simulink library "IO"  (R2025a)
settings: Solver=VariableStepAuto  StartTime=0.0  StopTime=10.0  RelTol=1e-3
values from neighbouring files (symbols this model uses):
  ADCBits = 12.0    [IO.sldd]
  Vref = 5.0    [IO.sldd]
undefined symbols (not defined in the file or in its folder): Bridge, dt, H, raptor_xcp_function
libraries: Raptor_lib x133, Utilities x20, Cooling x1
(part 2 of 6)

== system IO/CANOutputs/TCRegen ==
  IO_CAN2_154_Bus : Inport
  Bus Selector : BusSelector  OutputSignals=IO_RegenEnable_en,IO_TCActive_bool,IO_TCEnable_en,IO_TCSensitivity_en
  RollingCounterGenerator : Utilities/RollingCounterGenerator
  raptor_can_txmsg : Raptor_lib/CAN/raptor_can_txmsg  canDefinition=struct('dbcFile', 'SR26_CAN2.dbc','message', 'VCU_154','comment', '','signals', {{'VCU_counterMsg154','VCU_regenEnable','VCU_tCActive','VCU_tCEnable','VCU_tCSensitivity'}},'enabled', [ 1 1 1 1 1;],'scaled', [ 1 1 1 1 1;],'canBus', '''CAN2''','messageID', [ 154;],'idMask', [ 536870911;],'payloadMask', [],'payloadValue', [],'useDbcPeriod', [ 0;],'period', [ 100;],'queueSize', [ 1;],'label', [ 0;],'ver', [ 2;],'showID', [ 0;],'showRaw', [ 0;],'showRawMsg', [ 0;],'useStartVals', [ 0;],'extendedId', [ 0;],'useSimFunc', [ 0;],'sim_func_name', '''''','fill', [ 0;],'editID', [ 0;],'signalOrder', [ 1;],'signalAscDes', [ 1;],'msgLength', [ 8;])  canBus='CAN2'  queueSize=1  payloadMask=[]  payloadValue=[]  period=100  showID=0  label=0  idMask=hex2dec('1FFFFFFF')  fill=0  id=154  showRaw=0  signalOrder=1  signalInfo={{struct('Name', 'VCU_regenEnable','StartBit', [ 48;],'SignalSize', [ 8;],'ByteOrder', 'LittleEndian','ValueType', 'UNSIGNED','Class', 'uint8','Signed', [ 0;],'Factor', [ 1;],'Offset', [ 0;],'Min', [ 0;],'Max', [ 255;],'Units', '','StartVal', [ 0;],'Comment', 'Enumeration','Multiplexed', [ 0;],'Multiplexor', [ 0;],'MultiplexMode_Min', [],'MultiplexMode_Max', []),struct('Name', 'VCU_tCEnable','StartBit', [ 40;],'SignalSize', [ 8;],'ByteOrder', 'LittleEndian','ValueType', 'UNSIGNED','Class', 'uint8','Signed', [ 0;],'Factor', [ 1;],'Offset', [ 0;],'Min', [ 0;],'Max', [ 255;],'Units', '','StartVal', [ 0;],'Comment', 'Enumeration','Multiplexed', [ 0;],'Multiplexor', [ 0;],'MultiplexMode_Min', [],'MultiplexMode_Max', []),struct('Name', 'VCU_tCActive','StartBit', [ 32;],'SignalSize', [ 8;],'ByteOrder', 'LittleEndian','ValueType', 'UNSIGNED','Class', 'uint8','Signed', [ 0;],'Factor', [ 1;],'Offset', [ 0;],'Min', [ 0;],'Max', [ 255;],'Units', '','StartVal', [ 0;],'Comment', '0 = off, 1 = on Enumeration','Multiplexed', [ 0;],'Multiplexor', [ 0;],'MultiplexMode_Min', [],'MultiplexMode_Max', []),struct('Name', 'VCU_tCSensitivity','StartBit', [ 16;],'SignalSize', [ 16;],'ByteOrder', 'LittleEndian','ValueType', 'UNSIGNED','Class', 'uint16','Signed', [ 0;],'Factor', [ 1;],'Offset', [ 0;],'Min', [ -20;],'Max', [ 3276.7;],'Units', '','StartVal', [ 0;],'Comment', '','Multiplexed', [ 0;],'Multiplexor', [ 0;],'MultiplexMode_Min', [],'MultiplexMode_Max', []),struct('Name', 'VCU_counterMsg154','StartBit', [ 0;],'SignalSize', [ 4;],'ByteOrder', 'LittleEndian','ValueType', 'UNSIGNED','Class', 'uint8','Signed', [ 0;],'Factor', [ 1;],'Offset', [ 0;],'Min', [ 0;],'Max', [ 15;],'Units', '','StartVal', [ 0;],'Comment', 'Counter Message 154','Multiplexed', [ 0;],'Multiplexor', [ 0;],'MultiplexMode_Min', [],'MultiplexMode_Max', [])}}  useSimFunc=0  sim_func_name=''  useStartVals=0
      settings: SourceProductName=Raptor
  raptor_function_call_collector : Raptor_lib/Triggers/raptor_function_call_collector  count=10
      settings: SourceProductName=Raptor
  wires:
  Bus Selector/4 -> raptor_can_txmsg/5  "<IO_TCSensitivity_en>"
  Bus Selector/3 -> raptor_can_txmsg/4  "<IO_TCEnable_en>"
  Bus Selector/2 -> raptor_can_txmsg/3  "<IO_TCActive_bool>"
  Bus Selector/1 -> raptor_can_txmsg/2  "<IO_RegenEnable_en>"
  IO_CAN2_154_Bus/1 -> Bus Selector/1
  raptor_function_call_collector/1 -> RollingCounterGenerator/Trigger
  RollingCounterGenerator/1 -> raptor_can_txmsg/1

== system IO/CANOutputs/Throttle ==
  IO_CAN2_150_Bus : Inport
  Bus Selector : BusSelector  OutputSignals=IO_ThrottlePosition_pct,IO_ThrottlePosition1_pct,IO_ThrottlePosition2_pct
  RollingCounterGenerator : Utilities/RollingCounterGenerator
  raptor_can_txmsg : Raptor_lib/CAN/raptor_can_txmsg  canDefinition=struct('dbcFile', 'SR26_CAN2.dbc','message', 'VCU_150','comment', '','signals', {{'VCU_counterMsg150','VCU_throttlePosition','VCU_throttlePosition1','VCU_throttlePosition2'}},'enabled', [ 1 1 1 1;],'scaled', [ 1 1 1 1;],'canBus', '''CAN2''','messageID', [ 150;],'idMask', [ 536870911;],'payloadMask', [],'payloadValue', [],'useDbcPeriod', [ 0;],'period', [ 100;],'queueSize', [ 1;],'label', [ 0;],'ver', [ 2;],'showID', [ 0;],'showRaw', [ 0;],'showRawMsg', [ 0;],'useStartVals', [ 0;],'extendedId', [ 0;],'useSimFunc', [ 0;],'sim_func_name', '''''','fill', [ 0;],'editID', [ 0;],'signalOrder', [ 1;],'signalAscDes', [ 1;],'msgLength', [ 8;])  canBus='CAN2'  queueSize=1  payloadMask=[]  payloadValue=[]  period=100  showID=0  label=0  idMask=hex2dec('1FFFFFFF')  fill=0  id=150  showRaw=0  signalOrder=1  signalInfo={{struct('Name', 'VCU_throttlePosition2','StartBit', [ 48;],'SignalSize', [ 16;],'ByteOrder', 'LittleEndian','ValueType', 'SIGNED','Class', 'int16','Signed', [ 1;],'Factor', [ 0.1;],'Offset', [ 0;],'Min', [ 0;],'Max', [ 100;],'Units', '%','StartVal', [ 0;],'Comment', 'TPS2','Multiplexed', [ 0;],'Multiplexor', [ 0;],'MultiplexMode_Min', [],'MultiplexMode_Max', []),struct('Name', 'VCU_throttlePosition1','StartBit', [ 32;],'SignalSize', [ 16;],'ByteOrder', 'LittleEndian','ValueType', 'SIGNED','Class', 'int16','Signed', [ 1;],'Factor', [ 0.1;],'Offset', [ 0;],'Min', [ 0;],'Max', [ 100;],'Units', '%','StartVal', [ 0;],'Comment', 'TPS1','Multiplexed', [ 0;],'Multiplexor', [ 0;],'MultiplexMode_Min', [],'MultiplexMode_Max', []),struct('Name', 'VCU_throttlePosition','StartBit', [ 16;],'SignalSize', [ 16;],'ByteOrder', 'LittleEndian','ValueType', 'SIGNED','Class', 'int16','Signed', [ 1;],'Factor', [ 0.1;],'Offset', [ 0;],'Min', [ 0;],'Max', [ 100;],'Units', '%','StartVal', [ 0;],'Comment', 'Final throttle position','Multiplexed', [ 0;],'Multiplexor', [ 0;],'MultiplexMode_Min', [],'MultiplexMode_Max', []),struct('Name', 'VCU_counterMsg150','StartBit', [ 0;],'SignalSize', [ 4;],'ByteOrder', 'LittleEndian','ValueType', 'UNSIGNED','Class', 'uint8','Signed', [ 0;],'Factor', [ 1;],'Offset', [ 0;],'Min', [ 0;],'Max', [ 15;],'Units', '','StartVal', [ 0;],'Comment', 'Counter Message 150','Multiplexed', [ 0;],'Multiplexor', [ 0;],'MultiplexMode_Min', [],'MultiplexMode_Max', [])}}  useSimFunc=0  sim_func_name=''  useStartVals=0
      settings: SourceProductName=Raptor
  raptor_function_call_collector : Raptor_lib/Triggers/raptor_function_call_collector  count=10
      settings: SourceProductName=Raptor
  wires:
  IO_CAN2_150_Bus/1 -> Bus Selector/1
  Bus Selector/1 -> raptor_can_txmsg/2  "<IO_ThrottlePosition_pct>"
  Bus Selector/2 -> raptor_can_txmsg/3  "<IO_ThrottlePosition1_pct>"
  Bus Selector/3 -> raptor_can_txmsg/4  "<IO_ThrottlePosition2_pct>"
  RollingCounterGenerator/1 -> raptor_can_txmsg/1
  raptor_function_call_collector/1 -> RollingCounterGenerator/Trigger

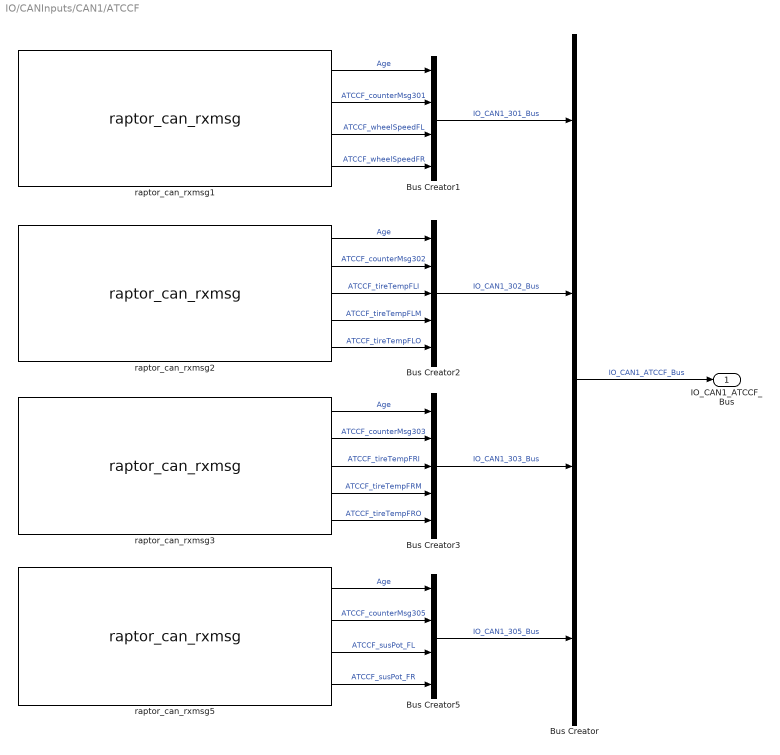
== system IO/CANInputs/CAN1/ATCCF ==
  Bus Creator : BusCreator  Inputs=4
  Bus Creator1 : BusCreator  Inputs=4
  Bus Creator2 : BusCreator  Inputs=5
  Bus Creator3 : BusCreator  Inputs=5
  Bus Creator5 : BusCreator  Inputs=4
  raptor_can_rxmsg1 : Raptor_lib/CAN/raptor_can_rxmsg  canDefinition=struct('dbcFile', 'SR26_CAN1.dbc','message', 'ATCCF_301','comment', '','signals', {{'ATCCF_counterMsg301','ATCCF_wheelSpeedFL','ATCCF_wheelSpeedFR'}},'enabled', [ 1 1 1;],'scaled', [ 1 1 1;],'canBus', '''CAN1''','messageID', [ 301;],'idMask', [ 536870911;],'payloadMask', [],'payloadValue', [],'period', [ 0;],'mailbox', '''''','queueSize', [ 1;],'label', [ 0;],'ver', [ 2;],'showID', [ 0;],'showRaw', [ 0;],'showRawMsg', [ 0;],'useStartVals', [ 0;],'extendedId', [ 0;],'showAge', [ 1;],'useSimFunc', [ 0;],'sim_func_name', '''''','fill', [ 0;],'editID', [ 0;],'signalOrder', [ 1;],'signalAscDes', [ 1;],'msgLength', [ 8;])  canBus='CAN1'  mailbox=''  payloadMask=[]  payloadValue=[]  idMask=hex2dec('1FFFFFFF')  queueSize=1  showID=0  label=0  fill=0  id=301  showRaw=0  showAge=1  signalOrder=1  signalInfo={{struct('Name', 'ATCCF_wheelSpeedFR','StartBit', [ 32;],'SignalSize', [ 16;],'ByteOrder', 'LittleEndian','ValueType', 'UNSIGNED','Class', 'uint16','Signed', [ 0;],'Factor', [ 1;],'Offset', [ 0;],'Min', [ 0;],'Max', [ 2000;],'Units', 'Hz','StartVal', [ 0;],'Comment', 'FR Angular Wheel Frequency','Multiplexed', [ 0;],'Multiplexor', [ 0;],'MultiplexMode_Min', [],'MultiplexMode_Max', []),struct('Name', 'ATCCF_wheelSpeedFL','StartBit', [ 16;],'SignalSize', [ 16;],'ByteOrder', 'LittleEndian','ValueType', 'UNSIGNED','Class', 'uint16','Signed', [ 0;],'Factor', [ 1;],'Offset', [ 0;],'Min', [ 0;],'Max', [ 2000;],'Units', 'Hz','StartVal', [ 0;],'Comment', 'FL Angular Wheel Frequency','Multiplexed', [ 0;],'Multiplexor', [ 0;],'MultiplexMode_Min', [],'MultiplexMode_Max', []),struct('Name', 'ATCCF_counterMsg301','StartBit', [ 0;],'SignalSize', [ 4;],'ByteOrder', 'LittleEndian','ValueType', 'UNSIGNED','Class', 'uint8','Signed', [ 0;],'Factor', [ 1;],'Offset', [ 0;],'Min', [ 0;],'Max', [ 15;],'Units', '','StartVal', [ 0;],'Comment', 'Counter Message 301','Multiplexed', [ 0;],'Multiplexor', [ 0;],'MultiplexMode_Min', [],'MultiplexMode_Max', [])}}  showRawMsg=0  useSimFunc=0  sim_func_name=''  useStartVals=0  extendedId=0
      settings: SourceProductName=Raptor
  raptor_can_rxmsg2 : Raptor_lib/CAN/raptor_can_rxmsg  canDefinition=struct('dbcFile', 'SR26_CAN1.dbc','message', 'ATCCF_302','comment', '','signals', {{'ATCCF_counterMsg302','ATCCF_tireTemp_FLI','ATCCF_tireTemp_FLM','ATCCF_tireTemp_FLO'}},'enabled', [ 1 1 1 1;],'scaled', [ 1 1 1 1;],'canBus', '''CAN1''','messageID', [ 302;],'idMask', [ 536870911;],'payloadMask', [],'payloadValue', [],'period', [ 0;],'mailbox', '''''','queueSize', [ 1;],'label', [ 0;],'ver', [ 2;],'showID', [ 0;],'showRaw', [ 0;],'showRawMsg', [ 0;],'useStartVals', [ 0;],'extendedId', [ 0;],'showAge', [ 1;],'useSimFunc', [ 0;],'sim_func_name', '''''','fill', [ 0;],'editID', [ 0;],'signalOrder', [ 1;],'signalAscDes', [ 1;],'msgLength', [ 8;])  canBus='CAN1'  mailbox=''  payloadMask=[]  payloadValue=[]  idMask=hex2dec('1FFFFFFF')  queueSize=1  showID=0  label=0  fill=0  id=302  showRaw=0  showAge=1  signalOrder=1  signalInfo={{struct('Name', 'ATCCF_tireTemp_FLI','StartBit', [ 48;],'SignalSize', [ 16;],'ByteOrder', 'LittleEndian','ValueType', 'SIGNED','Class', 'int16','Signed', [ 1;],'Factor', [ 1;],'Offset', [ 0;],'Min', [ 0;],'Max', [ 150;],'Units', 'degC','StartVal', [ 0;],'Comment', '','Multiplexed', [ 0;],'Multiplexor', [ 0;],'MultiplexMode_Min', [],'MultiplexMode_Max', []),struct('Name', 'ATCCF_tireTemp_FLM','StartBit', [ 32;],'SignalSize', [ 16;],'ByteOrder', 'LittleEndian','ValueType', 'SIGNED','Class', 'int16','Signed', [ 1;],'Factor', [ 1;],'Offset', [ 0;],'Min', [ 0;],'Max', [ 150;],'Units', 'degC','StartVal', [ 0;],'Comment', '','Multiplexed', [ 0;],'Multiplexor', [ 0;],'MultiplexMode_Min', [],'MultiplexMode_Max', []),struct('Name', 'ATCCF_tireTemp_FLO','StartBit', [ 16;],'SignalSize', [ 16;],'ByteOrder', 'LittleEndian','ValueType', 'SIGNED','Class', 'int16','Signed', [ 1;],'Factor', [ 1;],'Offset', [ 0;],'Min', [ 0;],'Max', [ 150;],'Units', 'degC','StartVal', [ 0;],'Comment', '','Multiplexed', [ 0;],'Multiplexor', [ 0;],'MultiplexMode_Min', [],'MultiplexMode_Max', []),struct('Name', 'ATCCF_counterMsg302','StartBit', [ 0;],'SignalSize', [ 4;],'ByteOrder', 'LittleEndian','ValueType', 'UNSIGNED','Class', 'uint8','Signed', [ 0;],'Factor', [ 1;],'Offset', [ 0;],'Min', [ 0;],'Max', [ 15;],'Units', '','StartVal', [ 0;],'Comment', '','Multiplexed', [ 0;],'Multiplexor', [ 0;],'MultiplexMode_Min', [],'MultiplexMode_Max', [])}}  showRawMsg=0  useSimFunc=0  sim_func_name=''  useStartVals=0  extendedId=0
      settings: SourceProductName=Raptor
  raptor_can_rxmsg3 : Raptor_lib/CAN/raptor_can_rxmsg  canDefinition=struct('dbcFile', 'SR26_CAN1.dbc','message', 'ATCCF_303','comment', '','signals', {{'ATCCF_counterMsg303','ATCCF_tireTemp_FRI','ATCCF_tireTemp_FRM','ATCCF_tireTemp_FRO'}},'enabled', [ 1 1 1 1;],'scaled', [ 1 1 1 1;],'canBus', '''CAN1''','messageID', [ 303;],'idMask', [ 536870911;],'payloadMask', [],'payloadValue', [],'period', [ 0;],'mailbox', '''''','queueSize', [ 1;],'label', [ 0;],'ver', [ 2;],'showID', [ 0;],'showRaw', [ 0;],'showRawMsg', [ 0;],'useStartVals', [ 0;],'extendedId', [ 0;],'showAge', [ 1;],'useSimFunc', [ 0;],'sim_func_name', '''''','fill', [ 0;],'editID', [ 0;],'signalOrder', [ 1;],'signalAscDes', [ 1;],'msgLength', [ 8;])  canBus='CAN1'  mailbox=''  payloadMask=[]  payloadValue=[]  idMask=hex2dec('1FFFFFFF')  queueSize=1  showID=0  label=0  fill=0  id=303  showRaw=0  showAge=1  signalOrder=1  signalInfo={{struct('Name', 'ATCCF_tireTemp_FRI','StartBit', [ 48;],'SignalSize', [ 16;],'ByteOrder', 'LittleEndian','ValueType', 'SIGNED','Class', 'int16','Signed', [ 1;],'Factor', [ 1;],'Offset', [ 0;],'Min', [ 0;],'Max', [ 150;],'Units', 'degC','StartVal', [ 0;],'Comment', '','Multiplexed', [ 0;],'Multiplexor', [ 0;],'MultiplexMode_Min', [],'MultiplexMode_Max', []),struct('Name', 'ATCCF_tireTemp_FRM','StartBit', [ 32;],'SignalSize', [ 16;],'ByteOrder', 'LittleEndian','ValueType', 'SIGNED','Class', 'int16','Signed', [ 1;],'Factor', [ 1;],'Offset', [ 0;],'Min', [ 0;],'Max', [ 150;],'Units', 'degC','StartVal', [ 0;],'Comment', '','Multiplexed', [ 0;],'Multiplexor', [ 0;],'MultiplexMode_Min', [],'MultiplexMode_Max', []),struct('Name', 'ATCCF_tireTemp_FRO','StartBit', [ 16;],'SignalSize', [ 16;],'ByteOrder', 'LittleEndian','ValueType', 'SIGNED','Class', 'int16','Signed', [ 1;],'Factor', [ 1;],'Offset', [ 0;],'Min', [ 0;],'Max', [ 150;],'Units', 'degC','StartVal', [ 0;],'Comment', '','Multiplexed', [ 0;],'Multiplexor', [ 0;],'MultiplexMode_Min', [],'MultiplexMode_Max', []),struct('Name', 'ATCCF_counterMsg303','StartBit', [ 0;],'SignalSize', [ 4;],'ByteOrder', 'LittleEndian','ValueType', 'UNSIGNED','Class', 'uint8','Signed', [ 0;],'Factor', [ 1;],'Offset', [ 0;],'Min', [ 0;],'Max', [ 15;],'Units', '','StartVal', [ 0;],'Comment', '','Multiplexed', [ 0;],'Multiplexor', [ 0;],'MultiplexMode_Min', [],'MultiplexMode_Max', [])}}  showRawMsg=0  useSimFunc=0  sim_func_name=''  useStartVals=0  extendedId=0
      settings: SourceProductName=Raptor
  raptor_can_rxmsg5 : Raptor_lib/CAN/raptor_can_rxmsg  canDefinition=struct('dbcFile', 'SR26_CAN1.dbc','message', 'ATCCF_305','comment', '','signals', {{'ATCCF_counterMsg305','ATCCF_susPot_FL','ATCCF_susPot_FR'}},'enabled', [ 1 1 1;],'scaled', [ 1 1 1;],'canBus', '''CAN1''','messageID', [ 305;],'idMask', [ 536870911;],'payloadMask', [],'payloadValue', [],'period', [ 0;],'mailbox', '''''','queueSize', [ 1;],'label', [ 0;],'ver', [ 2;],'showID', [ 0;],'showRaw', [ 0;],'showRawMsg', [ 0;],'useStartVals', [ 0;],'extendedId', [ 0;],'showAge', [ 1;],'useSimFunc', [ 0;],'sim_func_name', '''''','fill', [ 0;],'editID', [ 0;],'signalOrder', [ 1;],'signalAscDes', [ 1;],'msgLength', [ 8;])  canBus='CAN1'  mailbox=''  payloadMask=[]  payloadValue=[]  idMask=hex2dec('1FFFFFFF')  queueSize=1  showID=0  label=0  fill=0  id=305  showRaw=0  showAge=1  signalOrder=1  signalInfo={{struct('Name', 'ATCCF_susPot_FL','StartBit', [ 32;],'SignalSize', [ 16;],'ByteOrder', 'LittleEndian','ValueType', 'SIGNED','Class', 'int16','Signed', [ 1;],'Factor', [ 1;],'Offset', [ 0;],'Min', [ 0;],'Max', [ 500;],'Units', 'degC','StartVal', [ 0;],'Comment', '','Multiplexed', [ 0;],'Multiplexor', [ 0;],'MultiplexMode_Min', [],'MultiplexMode_Max', []),struct('Name', 'ATCCF_susPot_FR','StartBit', [ 16;],'SignalSize', [ 16;],'ByteOrder', 'LittleEndian','ValueType', 'SIGNED','Class', 'int16','Signed', [ 1;],'Factor', [ 1;],'Offset', [ 0;],'Min', [ 0;],'Max', [ 500;],'Units', 'degC','StartVal', [ 0;],'Comment', '','Multiplexed', [ 0;],'Multiplexor', [ 0;],'MultiplexMode_Min', [],'MultiplexMode_Max', []),struct('Name', 'ATCCF_counterMsg305','StartBit', [ 0;],'SignalSize', [ 4;],'ByteOrder', 'LittleEndian','ValueType', 'UNSIGNED','Class', 'uint8','Signed', [ 0;],'Factor', [ 1;],'Offset', [ 0;],'Min', [ 0;],'Max', [ 15;],'Units', '','StartVal', [ 0;],'Comment', '','Multiplexed', [ 0;],'Multiplexor', [ 0;],'MultiplexMode_Min', [],'MultiplexMode_Max', [])}}  showRawMsg=0  useSimFunc=0  sim_func_name=''  useStartVals=0  extendedId=0
      settings: SourceProductName=Raptor
  IO_CAN1_ATCCF_Bus : Outport
  wires:
  Bus Creator/1 -> IO_CAN1_ATCCF_Bus/1  "IO_CAN1_ATCCF_Bus"
  raptor_can_rxmsg5/1 -> Bus Creator5/1  "Age"
  raptor_can_rxmsg5/2 -> Bus Creator5/2  "ATCCF_counterMsg305"
  raptor_can_rxmsg5/3 -> Bus Creator5/3  "ATCCF_susPot_FL"
  raptor_can_rxmsg5/4 -> Bus Creator5/4  "ATCCF_susPot_FR"
  Bus Creator5/1 -> Bus Creator/4  "IO_CAN1_305_Bus"
  raptor_can_rxmsg3/1 -> Bus Creator3/1  "Age"
  raptor_can_rxmsg3/2 -> Bus Creator3/2  "ATCCF_counterMsg303"
  raptor_can_rxmsg3/3 -> Bus Creator3/3  "ATCCF_tireTempFRI"
  raptor_can_rxmsg3/4 -> Bus Creator3/4  "ATCCF_tireTempFRM"
  Bus Creator3/1 -> Bus Creator/3  "IO_CAN1_303_Bus"
  raptor_can_rxmsg3/5 -> Bus Creator3/5  "ATCCF_tireTempFRO"
  raptor_can_rxmsg2/5 -> Bus Creator2/5  "ATCCF_tireTempFLO"
  Bus Creator2/1 -> Bus Creator/2  "IO_CAN1_302_Bus"
  raptor_can_rxmsg2/4 -> Bus Creator2/4  "ATCCF_tireTempFLM"
  raptor_can_rxmsg2/3 -> Bus Creator2/3  "ATCCF_tireTempFLI"
  raptor_can_rxmsg2/2 -> Bus Creator2/2  "ATCCF_counterMsg302"
  raptor_can_rxmsg2/1 -> Bus Creator2/1  "Age"
  raptor_can_rxmsg1/1 -> Bus Creator1/1  "Age"
  raptor_can_rxmsg1/2 -> Bus Creator1/2  "ATCCF_counterMsg301"
  raptor_can_rxmsg1/3 -> Bus Creator1/3  "ATCCF_wheelSpeedFL"
  raptor_can_rxmsg1/4 -> Bus Creator1/4  "ATCCF_wheelSpeedFR"
  Bus Creator1/1 -> Bus Creator/1  "IO_CAN1_301_Bus"

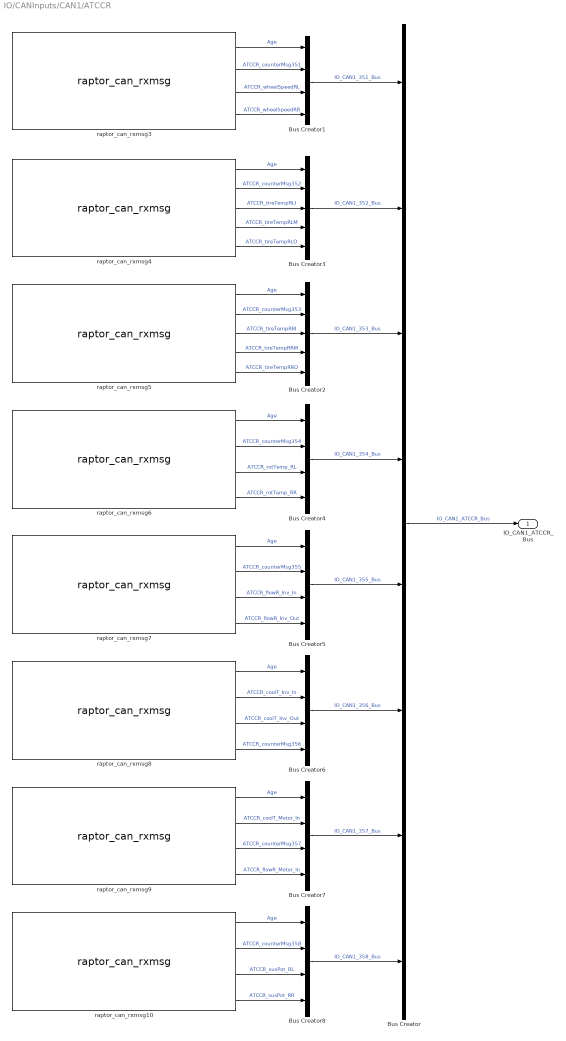
== system IO/CANInputs/CAN1/ATCCR ==
  Bus Creator : BusCreator  Inputs=8
  Bus Creator{1,4..8} (6 alike) : BusCreator  Inputs=4
  Bus Creator2 : BusCreator  Inputs=5
  Bus Creator3 : BusCreator  Inputs=5
  raptor_can_rxmsg10 : Raptor_lib/CAN/raptor_can_rxmsg  canDefinition=struct('dbcFile', 'SR26_CAN1.dbc','message', 'ATCCR_358','comment', '','signals', {{'ATCCR_counterMsg358','ATCCR_susPot_RL','ATCCR_susPot_RR'}},'enabled', [ 1 1 1;],'scaled', [ 1 1 1;],'canBus', '''CAN1''','messageID', [ 358;],'idMask', [ 536870911;],'payloadMask', [],'payloadValue', [],'period', [ 0;],'mailbox', '''''','queueSize', [ 1;],'label', [ 0;],'ver', [ 2;],'showID', [ 0;],'showRaw', [ 0;],'showRawMsg', [ 0;],'useStartVals', [ 0;],'extendedId', [ 0;],'showAge', [ 1;],'useSimFunc', [ 0;],'sim_func_name', '''''','fill', [ 0;],'editID', [ 0;],'signalOrder', [ 1;],'signalAscDes', [ 1;],'msgLength', [ 8;])  canBus='CAN1'  mailbox=''  payloadMask=[]  payloadValue=[]  idMask=hex2dec('1FFFFFFF')  queueSize=1  showID=0  label=0  fill=0  id=358  showRaw=0  showAge=1  signalOrder=1  signalInfo={{struct('Name', 'ATCCR_susPot_RR','StartBit', [ 32;],'SignalSize', [ 16;],'ByteOrder', 'LittleEndian','ValueType', 'SIGNED','Class', 'int16','Signed', [ 1;],'Factor', [ 1;],'Offset', [ 0;],'Min', [ 0;],'Max', [ 500;],'Units', 'degC','StartVal', [ 0;],'Comment', '','Multiplexed', [ 0;],'Multiplexor', [ 0;],'MultiplexMode_Min', [],'MultiplexMode_Max', []),struct('Name', 'ATCCR_susPot_RL','StartBit', [ 16;],'SignalSize', [ 16;],'ByteOrder', 'LittleEndian','ValueType', 'SIGNED','Class', 'int16','Signed', [ 1;],'Factor', [ 1;],'Offset', [ 0;],'Min', [ 0;],'Max', [ 500;],'Units', 'degC','StartVal', [ 0;],'Comment', '','Multiplexed', [ 0;],'Multiplexor', [ 0;],'MultiplexMode_Min', [],'MultiplexMode_Max', []),struct('Name', 'ATCCR_counterMsg358','StartBit', [ 0;],'SignalSize', [ 4;],'ByteOrder', 'LittleEndian','ValueType', 'UNSIGNED','Class', 'uint8','Signed', [ 0;],'Factor', [ 1;],'Offset', [ 0;],'Min', [ 0;],'Max', [ 15;],'Units', '','StartVal', [ 0;],'Comment', '','Multiplexed', [ 0;],'Multiplexor', [ 0;],'MultiplexMode_Min', [],'MultiplexMode_Max', [])}}  showRawMsg=0  useSimFunc=0  sim_func_name=''  useStartVals=0  extendedId=0
      settings: SourceProductName=Raptor
  raptor_can_rxmsg3 : Raptor_lib/CAN/raptor_can_rxmsg  canDefinition=struct('dbcFile', 'SR26_CAN1.dbc','message', 'ATCCR_351','comment', '','signals', {{'ATCCR_counterMsg351','ATCCR_wheelSpeedRL','ATCCR_wheelSpeedRR'}},'enabled', [ 1 1 1;],'scaled', [ 1 1 1;],'canBus', '''CAN1''','messageID', [ 351;],'idMask', [ 536870911;],'payloadMask', [],'payloadValue', [],'period', [ 0;],'mailbox', '''''','queueSize', [ 1;],'label', [ 0;],'ver', [ 2;],'showID', [ 0;],'showRaw', [ 0;],'showRawMsg', [ 0;],'useStartVals', [ 0;],'extendedId', [ 0;],'showAge', [ 1;],'useSimFunc', [ 0;],'sim_func_name', '''''','fill', [ 0;],'editID', [ 0;],'signalOrder', [ 1;],'signalAscDes', [ 1;],'msgLength', [ 8;])  canBus='CAN1'  mailbox=''  payloadMask=[]  payloadValue=[]  idMask=hex2dec('1FFFFFFF')  queueSize=1  showID=0  label=0  fill=0  id=351  showRaw=0  showAge=1  signalOrder=1  signalInfo={{struct('Name', 'ATCCR_wheelSpeedRR','StartBit', [ 32;],'SignalSize', [ 16;],'ByteOrder', 'LittleEndian','ValueType', 'UNSIGNED','Class', 'uint16','Signed', [ 0;],'Factor', [ 1;],'Offset', [ 0;],'Min', [ 0;],'Max', [ 2000;],'Units', 'Hz','StartVal', [ 0;],'Comment', 'FR Angular Wheel Frequency','Multiplexed', [ 0;],'Multiplexor', [ 0;],'MultiplexMode_Min', [],'MultiplexMode_Max', []),struct('Name', 'ATCCR_wheelSpeedRL','StartBit', [ 16;],'SignalSize', [ 16;],'ByteOrder', 'LittleEndian','ValueType', 'UNSIGNED','Class', 'uint16','Signed', [ 0;],'Factor', [ 1;],'Offset', [ 0;],'Min', [ 0;],'Max', [ 2000;],'Units', 'Hz','StartVal', [ 0;],'Comment', 'FL Angular Wheel Frequency','Multiplexed', [ 0;],'Multiplexor', [ 0;],'MultiplexMode_Min', [],'MultiplexMode_Max', []),struct('Name', 'ATCCR_counterMsg351','StartBit', [ 0;],'SignalSize', [ 4;],'ByteOrder', 'LittleEndian','ValueType', 'UNSIGNED','Class', 'uint8','Signed', [ 0;],'Factor', [ 1;],'Offset', [ 0;],'Min', [ 0;],'Max', [ 15;],'Units', '','StartVal', [ 0;],'Comment', 'Counter Message 351','Multiplexed', [ 0;],'Multiplexor', [ 0;],'MultiplexMode_Min', [],'MultiplexMode_Max', [])}}  showRawMsg=0  useSimFunc=0  sim_func_name=''  useStartVals=0  extendedId=0
      settings: SourceProductName=Raptor
  raptor_can_rxmsg4 : Raptor_lib/CAN/raptor_can_rxmsg  canDefinition=struct('dbcFile', 'SR26_CAN1.dbc','message', 'ATCCR_352','comment', '','signals', {{'ATCCR_counterMsg352','ATCCR_tireTemp_RLI','ATCCR_tireTemp_RLM','ATCCR_tireTemp_RLO'}},'enabled', [ 1 1 1 1;],'scaled', [ 1 1 1 1;],'canBus', '''CAN1''','messageID', [ 352;],'idMask', [ 536870911;],'payloadMask', [],'payloadValue', [],'period', [ 0;],'mailbox', '''''','queueSize', [ 1;],'label', [ 0;],'ver', [ 2;],'showID', [ 0;],'showRaw', [ 0;],'showRawMsg', [ 0;],'useStartVals', [ 0;],'extendedId', [ 0;],'showAge', [ 1;],'useSimFunc', [ 0;],'sim_func_name', '''''','fill', [ 0;],'editID', [ 0;],'signalOrder', [ 1;],'signalAscDes', [ 1;],'msgLength', [ 8;])  canBus='CAN1'  mailbox=''  payloadMask=[]  payloadValue=[]  idMask=hex2dec('1FFFFFFF')  queueSize=1  showID=0  label=0  fill=0  id=352  showRaw=0  showAge=1  signalOrder=1  signalInfo={{struct('Name', 'ATCCR_tireTemp_RLI','StartBit', [ 48;],'SignalSize', [ 16;],'ByteOrder', 'LittleEndian','ValueType', 'SIGNED','Class', 'int16','Signed', [ 1;],'Factor', [ 1;],'Offset', [ 0;],'Min', [ 0;],'Max', [ 150;],'Units', 'degC','StartVal', [ 0;],'Comment', '','Multiplexed', [ 0;],'Multiplexor', [ 0;],'MultiplexMode_Min', [],'MultiplexMode_Max', []),struct('Name', 'ATCCR_tireTemp_RLM','StartBit', [ 32;],'SignalSize', [ 16;],'ByteOrder', 'LittleEndian','ValueType', 'SIGNED','Class', 'int16','Signed', [ 1;],'Factor', [ 1;],'Offset', [ 0;],'Min', [ 0;],'Max', [ 150;],'Units', 'degC','StartVal', [ 0;],'Comment', '','Multiplexed', [ 0;],'Multiplexor', [ 0;],'MultiplexMode_Min', [],'MultiplexMode_Max', []),struct('Name', 'ATCCR_tireTemp_RLO','StartBit', [ 16;],'SignalSize', [ 16;],'ByteOrder', 'LittleEndian','ValueType', 'SIGNED','Class', 'int16','Signed', [ 1;],'Factor', [ 1;],'Offset', [ 0;],'Min', [ 0;],'Max', [ 150;],'Units', 'degC','StartVal', [ 0;],'Comment', '','Multiplexed', [ 0;],'Multiplexor', [ 0;],'MultiplexMode_Min', [],'MultiplexMode_Max', []),struct('Name', 'ATCCR_counterMsg352','StartBit', [ 0;],'SignalSize', [ 4;],'ByteOrder', 'LittleEndian','ValueType', 'UNSIGNED','Class', 'uint8','Signed', [ 0;],'Factor', [ 1;],'Offset', [ 0;],'Min', [ 0;],'Max', [ 15;],'Units', '','StartVal', [ 0;],'Comment', '','Multiplexed', [ 0;],'Multiplexor', [ 0;],'MultiplexMode_Min', [],'MultiplexMode_Max', [])}}  showRawMsg=0  useSimFunc=0  sim_func_name=''  useStartVals=0  extendedId=0
      settings: SourceProductName=Raptor
  raptor_can_rxmsg5 : Raptor_lib/CAN/raptor_can_rxmsg  canDefinition=struct('dbcFile', 'SR26_CAN1.dbc','message', 'ATCCR_353','comment', '','signals', {{'ATCCR_counterMsg353','ATCCR_tireTemp_RRI','ATCCR_tireTemp_RRM','ATCCR_tireTemp_RRO'}},'enabled', [ 1 1 1 1;],'scaled', [ 1 1 1 1;],'canBus', '''CAN1''','messageID', [ 353;],'idMask', [ 536870911;],'payloadMask', [],'payloadValue', [],'period', [ 0;],'mailbox', '''''','queueSize', [ 1;],'label', [ 0;],'ver', [ 2;],'showID', [ 0;],'showRaw', [ 0;],'showRawMsg', [ 0;],'useStartVals', [ 0;],'extendedId', [ 0;],'showAge', [ 1;],'useSimFunc', [ 0;],'sim_func_name', '''''','fill', [ 0;],'editID', [ 0;],'signalOrder', [ 1;],'signalAscDes', [ 1;],'msgLength', [ 8;])  canBus='CAN1'  mailbox=''  payloadMask=[]  payloadValue=[]  idMask=hex2dec('1FFFFFFF')  queueSize=1  showID=0  label=0  fill=0  id=353  showRaw=0  showAge=1  signalOrder=1  signalInfo={{struct('Name', 'ATCCR_tireTemp_RRI','StartBit', [ 48;],'SignalSize', [ 16;],'ByteOrder', 'LittleEndian','ValueType', 'SIGNED','Class', 'int16','Signed', [ 1;],'Factor', [ 1;],'Offset', [ 0;],'Min', [ 0;],'Max', [ 150;],'Units', 'degC','StartVal', [ 0;],'Comment', '','Multiplexed', [ 0;],'Multiplexor', [ 0;],'MultiplexMode_Min', [],'MultiplexMode_Max', []),struct('Name', 'ATCCR_tireTemp_RRM','StartBit', [ 32;],'SignalSize', [ 16;],'ByteOrder', 'LittleEndian','ValueType', 'SIGNED','Class', 'int16','Signed', [ 1;],'Factor', [ 1;],'Offset', [ 0;],'Min', [ 0;],'Max', [ 150;],'Units', 'degC','StartVal', [ 0;],'Comment', '','Multiplexed', [ 0;],'Multiplexor', [ 0;],'MultiplexMode_Min', [],'MultiplexMode_Max', []),struct('Name', 'ATCCR_tireTemp_RRO','StartBit', [ 16;],'SignalSize', [ 16;],'ByteOrder', 'LittleEndian','ValueType', 'SIGNED','Class', 'int16','Signed', [ 1;],'Factor', [ 1;],'Offset', [ 0;],'Min', [ 0;],'Max', [ 150;],'Units', 'degC','StartVal', [ 0;],'Comment', '','Multiplexed', [ 0;],'Multiplexor', [ 0;],'MultiplexMode_Min', [],'MultiplexMode_Max', []),struct('Name', 'ATCCR_counterMsg353','StartBit', [ 0;],'SignalSize', [ 4;],'ByteOrder', 'LittleEndian','ValueType', 'UNSIGNED','Class', 'uint8','Signed', [ 0;],'Factor', [ 1;],'Offset', [ 0;],'Min', [ 0;],'Max', [ 15;],'Units', '','StartVal', [ 0;],'Comment', '','Multiplexed', [ 0;],'Multiplexor', [ 0;],'MultiplexMode_Min', [],'MultiplexMode_Max', [])}}  showRawMsg=0  useSimFunc=0  sim_func_name=''  useStartVals=0  extendedId=0
      settings: SourceProductName=Raptor
  raptor_can_rxmsg6 : Raptor_lib/CAN/raptor_can_rxmsg  canDefinition=struct('dbcFile', 'SR26_CAN1.dbc','message', 'ATCCR_354','comment', '','signals', {{'ATCCR_counterMsg354','ATCCR_rotTemp_RL','ATCCR_rotTemp_RR'}},'enabled', [ 1 1 1;],'scaled', [ 1 1 1;],'canBus', '''CAN1''','messageID', [ 354;],'idMask', [ 536870911;],'payloadMask', [],'payloadValue', [],'period', [ 0;],'mailbox', '''''','queueSize', [ 1;],'label', [ 0;],'ver', [ 2;],'showID', [ 0;],'showRaw', [ 0;],'showRawMsg', [ 0;],'useStartVals', [ 0;],'extendedId', [ 0;],'showAge', [ 1;],'useSimFunc', [ 0;],'sim_func_name', '''''','fill', [ 0;],'editID', [ 0;],'signalOrder', [ 1;],'signalAscDes', [ 1;],'msgLength', [ 8;])  canBus='CAN1'  mailbox=''  payloadMask=[]  payloadValue=[]  idMask=hex2dec('1FFFFFFF')  queueSize=1  showID=0  label=0  fill=0  id=354  showRaw=0  showAge=1  signalOrder=1  signalInfo={{struct('Name', 'ATCCR_rotTemp_RR','StartBit', [ 32;],'SignalSize', [ 16;],'ByteOrder', 'LittleEndian','ValueType', 'SIGNED','Class', 'int16','Signed', [ 1;],'Factor', [ 1;],'Offset', [ 0;],'Min', [ 0;],'Max', [ 500;],'Units', 'degC','StartVal', [ 0;],'Comment', '','Multiplexed', [ 0;],'Multiplexor', [ 0;],'MultiplexMode_Min', [],'MultiplexMode_Max', []),struct('Name', 'ATCCR_rotTemp_RL','StartBit', [ 16;],'SignalSize', [ 16;],'ByteOrder', 'LittleEndian','ValueType', 'SIGNED','Class', 'int16','Signed', [ 1;],'Factor', [ 1;],'Offset', [ 0;],'Min', [ 0;],'Max', [ 500;],'Units', 'degC','StartVal', [ 0;],'Comment', '','Multiplexed', [ 0;],'Multiplexor', [ 0;],'MultiplexMode_Min', [],'MultiplexMode_Max', []),struct('Name', 'ATCCR_counterMsg354','StartBit', [ 0;],'SignalSize', [ 4;],'ByteOrder', 'LittleEndian','ValueType', 'UNSIGNED','Class', 'uint8','Signed', [ 0;],'Factor', [ 1;],'Offset', [ 0;],'Min', [ 0;],'Max', [ 15;],'Units', '','StartVal', [ 0;],'Comment', '','Multiplexed', [ 0;],'Multiplexor', [ 0;],'MultiplexMode_Min', [],'MultiplexMode_Max', [])}}  showRawMsg=0  useSimFunc=0  sim_func_name=''  useStartVals=0  extendedId=0
      settings: SourceProductName=Raptor
  raptor_can_rxmsg7 : Raptor_lib/CAN/raptor_can_rxmsg  canDefinition=struct('dbcFile', 'SR26_CAN1.dbc','message', 'ATCCR_355','comment', '','signals', {{'ATCCR_counterMsg355','ATCCR_flowR_Inv_In','ATCCR_flowR_Inv_Out'}},'enabled', [ 1 1 1;],'scaled', [ 1 1 1;],'canBus', '''CAN1''','messageID', [ 355;],'idMask', [ 536870911;],'payloadMask', [],'payloadValue', [],'period', [ 0;],'mailbox', '''''','queueSize', [ 1;],'label', [ 0;],'ver', [ 2;],'showID', [ 0;],'showRaw', [ 0;],'showRawMsg', [ 0;],'useStartVals', [ 0;],'extendedId', [ 0;],'showAge', [ 1;],'useSimFunc', [ 0;],'sim_func_name', '''''','fill', [ 0;],'editID', [ 0;],'signalOrder', [ 1;],'signalAscDes', [ 1;],'msgLength', [ 8;])  canBus='CAN1'  mailbox=''  payloadMask=[]  payloadValue=[]  idMask=hex2dec('1FFFFFFF')  queueSize=1  showID=0  label=0  fill=0  id=355  showRaw=0  showAge=1  signalOrder=1  signalInfo={{struct('Name', 'ATCCR_flowR_Inv_Out','StartBit', [ 32;],'SignalSize', [ 16;],'ByteOrder', 'LittleEndian','ValueType', 'SIGNED','Class', 'int16','Signed', [ 1;],'Factor', [ 1;],'Offset', [ 0;],'Min', [ 0;],'Max', [ 150;],'Units', 'degC','StartVal', [ 0;],'Comment', '','Multiplexed', [ 0;],'Multiplexor', [ 0;],'MultiplexMode_Min', [],'MultiplexMode_Max', []),struct('Name', 'ATCCR_flowR_Inv_In','StartBit', [ 16;],'SignalSize', [ 16;],'ByteOrder', 'LittleEndian','ValueType', 'SIGNED','Class', 'int16','Signed', [ 1;],'Factor', [ 1;],'Offset', [ 0;],'Min', [ 0;],'Max', [ 150;],'Units', 'degC','StartVal', [ 0;],'Comment', '','Multiplexed', [ 0;],'Multiplexor', [ 0;],'MultiplexMode_Min', [],'MultiplexMode_Max', []),struct('Name', 'ATCCR_counterMsg355','StartBit', [ 0;],'SignalSize', [ 4;],'ByteOrder', 'LittleEndian','ValueType', 'UNSIGNED','Class', 'uint8','Signed', [ 0;],'Factor', [ 1;],'Offset', [ 0;],'Min', [ 0;],'Max', [ 15;],'Units', '','StartVal', [ 0;],'Comment', '','Multiplexed', [ 0;],'Multiplexor', [ 0;],'MultiplexMode_Min', [],'MultiplexMode_Max', [])}}  showRawMsg=0  useSimFunc=0  sim_func_name=''  useStartVals=0  extendedId=0
      settings: SourceProductName=Raptor
  raptor_can_rxmsg8 : Raptor_lib/CAN/raptor_can_rxmsg  canDefinition=struct('dbcFile', 'SR26_CAN1.dbc','message', 'ATCCR_356','comment', '','signals', {{'ATCCR_coolT_Inv_In','ATCCR_coolT_Inv_Out','ATCCR_counterMsg356'}},'enabled', [ 1 1 1;],'scaled', [ 1 1 1;],'canBus', '''CAN1''','messageID', [ 356;],'idMask', [ 536870911;],'payloadMask', [],'payloadValue', [],'period', [ 0;],'mailbox', '''''','queueSize', [ 1;],'label', [ 0;],'ver', [ 2;],'showID', [ 0;],'showRaw', [ 0;],'showRawMsg', [ 0;],'useStartVals', [ 0;],'extendedId', [ 0;],'showAge', [ 1;],'useSimFunc', [ 0;],'sim_func_name', '''''','fill', [ 0;],'editID', [ 0;],'signalOrder', [ 1;],'signalAscDes', [ 1;],'msgLength', [ 8;])  canBus='CAN1'  mailbox=''  payloadMask=[]  payloadValue=[]  idMask=hex2dec('1FFFFFFF')  queueSize=1  showID=0  label=0  fill=0  id=356  showRaw=0  showAge=1  signalOrder=1  signalInfo={{struct('Name', 'ATCCR_coolT_Inv_Out','StartBit', [ 32;],'SignalSize', [ 16;],'ByteOrder', 'LittleEndian','ValueType', 'SIGNED','Class', 'int16','Signed', [ 1;],'Factor', [ 1;],'Offset', [ 0;],'Min', [ 0;],'Max', [ 150;],'Units', 'degC','StartVal', [ 0;],'Comment', '','Multiplexed', [ 0;],'Multiplexor', [ 0;],'MultiplexMode_Min', [],'MultiplexMode_Max', []),struct('Name', 'ATCCR_coolT_Inv_In','StartBit', [ 16;],'SignalSize', [ 16;],'ByteOrder', 'LittleEndian','ValueType', 'SIGNED','Class', 'int16','Signed', [ 1;],'Factor', [ 1;],'Offset', [ 0;],'Min', [ 0;],'Max', [ 150;],'Units', 'degC','StartVal', [ 0;],'Comment', '','Multiplexed', [ 0;],'Multiplexor', [ 0;],'MultiplexMode_Min', [],'MultiplexMode_Max', []),struct('Name', 'ATCCR_counterMsg356','StartBit', [ 0;],'SignalSize', [ 4;],'ByteOrder', 'LittleEndian','ValueType', 'UNSIGNED','Class', 'uint8','Signed', [ 0;],'Factor', [ 1;],'Offset', [ 0;],'Min', [ 0;],'Max', [ 15;],'Units', '','StartVal', [ 0;],'Comment', '','Multiplexed', [ 0;],'Multiplexor', [ 0;],'MultiplexMode_Min', [],'MultiplexMode_Max', [])}}  showRawMsg=0  useSimFunc=0  sim_func_name=''  useStartVals=0  extendedId=0
      settings: SourceProductName=Raptor
  raptor_can_rxmsg9 : Raptor_lib/CAN/raptor_can_rxmsg  canDefinition=struct('dbcFile', 'SR26_CAN1.dbc','message', 'ATCCR_357','comment', '','signals', {{'ATCCR_coolT_Motor_In','ATCCR_counterMsg357','ATCCR_flowR_Motor_In'}},'enabled', [ 1 1 1;],'scaled', [ 1 1 1;],'canBus', '''CAN1''','messageID', [ 357;],'idMask', [ 536870911;],'payloadMask', [],'payloadValue', [],'period', [ 0;],'mailbox', '''''','queueSize', [ 1;],'label', [ 0;],'ver', [ 2;],'showID', [ 0;],'showRaw', [ 0;],'showRawMsg', [ 0;],'useStartVals', [ 0;],'extendedId', [ 0;],'showAge', [ 1;],'useSimFunc', [ 0;],'sim_func_name', '''''','fill', [ 0;],'editID', [ 0;],'signalOrder', [ 1;],'signalAscDes', [ 1;],'msgLength', [ 8;])  canBus='CAN1'  mailbox=''  payloadMask=[]  payloadValue=[]  idMask=hex2dec('1FFFFFFF')  queueSize=1  showID=0  label=0  fill=0  id=357  showRaw=0  showAge=1  signalOrder=1  signalInfo={{struct('Name', 'ATCCR_coolT_Motor_In','StartBit', [ 32;],'SignalSize', [ 16;],'ByteOrder', 'LittleEndian','ValueType', 'SIGNED','Class', 'int16','Signed', [ 1;],'Factor', [ 1;],'Offset', [ 0;],'Min', [ 0;],'Max', [ 150;],'Units', 'degC','StartVal', [ 0;],'Comment', '','Multiplexed', [ 0;],'Multiplexor', [ 0;],'MultiplexMode_Min', [],'MultiplexMode_Max', []),struct('Name', 'ATCCR_flowR_Motor_In','StartBit', [ 16;],'SignalSize', [ 16;],'ByteOrder', 'LittleEndian','ValueType', 'SIGNED','Class', 'int16','Signed', [ 1;],'Factor', [ 1;],'Offset', [ 0;],'Min', [ 0;],'Max', [ 150;],'Units', 'degC','StartVal', [ 0;],'Comment', '','Multiplexed', [ 0;],'Multiplexor', [ 0;],'MultiplexMode_Min', [],'MultiplexMode_Max', []),struct('Name', 'ATCCR_counterMsg357','StartBit', [ 0;],'SignalSize', [ 4;],'ByteOrder', 'LittleEndian','ValueType', 'UNSIGNED','Class', 'uint8','Signed', [ 0;],'Factor', [ 1;],'Offset', [ 0;],'Min', [ 0;],'Max', [ 15;],'Units', '','StartVal', [ 0;],'Comment', '','Multiplexed', [ 0;],'Multiplexor', [ 0;],'MultiplexMode_Min', [],'MultiplexMode_Max', [])}}  showRawMsg=0  useSimFunc=0  sim_func_name=''  useStartVals=0  extendedId=0
      settings: SourceProductName=Raptor
  IO_CAN1_ATCCR_Bus : Outport
  wires:
  raptor_can_rxmsg7/2 -> Bus Creator5/2  "ATCCR_counterMsg355"
  Bus Creator5/1 -> Bus Creator/5  "IO_CAN1_355_Bus"
  Bus Creator3/1 -> Bus Creator/2  "IO_CAN1_352_Bus"
  raptor_can_rxmsg3/4 -> Bus Creator1/4  "ATCCR_wheelSpeedRR"
  Bus Creator7/1 -> Bus Creator/7  "IO_CAN1_357_Bus"
  raptor_can_rxmsg8/2 -> Bus Creator6/2  "ATCCR_coolT_Inv_In"
  Bus Creator4/1 -> Bus Creator/4  "IO_CAN1_354_Bus"
  Bus Creator1/1 -> Bus Creator/1  "IO_CAN1_351_Bus"
  Bus Creator/1 -> IO_CAN1_ATCCR_Bus/1  "IO_CAN1_ATCCR_Bus"
  raptor_can_rxmsg7/1 -> Bus Creator5/1  "Age"
  raptor_can_rxmsg5/3 -> Bus Creator2/3  "ATCCR_tireTempRRI"
  Bus Creator6/1 -> Bus Creator/6  "IO_CAN1_356_Bus"
  Bus Creator8/1 -> Bus Creator/8  "IO_CAN1_358_Bus"
  Bus Creator2/1 -> Bus Creator/3  "IO_CAN1_353_Bus"
  raptor_can_rxmsg5/2 -> Bus Creator2/2  "ATCCR_counterMsg353"
  raptor_can_rxmsg7/3 -> Bus Creator5/3  "ATCCR_flowR_Inv_In"
  raptor_can_rxmsg5/4 -> Bus Creator2/4  "ATCCR_tireTempRRM"
  raptor_can_rxmsg4/3 -> Bus Creator3/3  "ATCCR_tireTempRLI"
  raptor_can_rxmsg5/1 -> Bus Creator2/1  "Age"
  raptor_can_rxmsg5/5 -> Bus Creator2/5  "ATCCR_tireTempRRO"
  raptor_can_rxmsg6/3 -> Bus Creator4/3  "ATCCR_rotTemp_RL"
  raptor_can_rxmsg10/3 -> Bus Creator8/3  "ATCCR_susPot_RL"
  raptor_can_rxmsg6/4 -> Bus Creator4/4  "ATCCR_rotTemp_RR"
  raptor_can_rxmsg6/2 -> Bus Creator4/2  "ATCCR_counterMsg354"
  raptor_can_rxmsg10/2 -> Bus Creator8/2  "ATCCR_counterMsg358"
  raptor_can_rxmsg10/4 -> Bus Creator8/4  "ATCCR_susPot_RR"
  raptor_can_rxmsg10/1 -> Bus Creator8/1  "Age"
  raptor_can_rxmsg4/1 -> Bus Creator3/1  "Age"
  raptor_can_rxmsg9/3 -> Bus Creator7/3  "ATCCR_counterMsg357"
  raptor_can_rxmsg9/4 -> Bus Creator7/4  "ATCCR_flowR_Motor_In"
  raptor_can_rxmsg8/3 -> Bus Creator6/3  "ATCCR_coolT_Inv_Out"
  raptor_can_rxmsg9/2 -> Bus Creator7/2  "ATCCR_coolT_Motor_In"
  raptor_can_rxmsg9/1 -> Bus Creator7/1  "Age"
  raptor_can_rxmsg4/5 -> Bus Creator3/5  "ATCCR_tireTempRLO"
  raptor_can_rxmsg4/2 -> Bus Creator3/2  "ATCCR_counterMsg352"
  raptor_can_rxmsg4/4 -> Bus Creator3/4  "ATCCR_tireTempRLM"
  raptor_can_rxmsg3/2 -> Bus Creator1/2  "ATCCR_counterMsg351"
  raptor_can_rxmsg3/3 -> Bus Creator1/3  "ATCCR_wheelSpeedRL"
  raptor_can_rxmsg3/1 -> Bus Creator1/1  "Age"
  raptor_can_rxmsg7/4 -> Bus Creator5/4  "ATCCR_flowR_Inv_Out"
  raptor_can_rxmsg6/1 -> Bus Creator4/1  "Age"
  raptor_can_rxmsg8/1 -> Bus Creator6/1  "Age"
  raptor_can_rxmsg8/4 -> Bus Creator6/4  "ATCCR_counterMsg356"

== system IO/CANInputs/CAN1/DCDC ==
  Bus Creator1 : BusCreator  Inputs=19
  raptor_can_rxmsg3 : Raptor_lib/CAN/raptor_can_rxmsg  canDefinition=struct('dbcFile', 'SR26_CAN1.dbc','message', 'DCDC_1801D08F','comment', '','signals', {{'DCDC_canError','DCDC_currentOutput','DCDC_fanControl1','DCDC_fanControl2','DCDC_hardwareFault','DCDC_hvilError','DCDC_inputOverVoltage','DCDC_inputUnderVoltage','DCDC_outputOverCurrent','DCDC_outputOverVoltage','DCDC_outputUnderVoltage','DCDC_overTempError','DCDC_ready','DCDC_shutOffError','DCDC_status','DCDC_tempWarning','DCDC_temperature','DCDC_voltageOutput'}},'enabled', [ 1 1 1 1 1 1 1 1 1 1 1 1 1 1 1 1 1 1;],'scaled', [ 1 1 1 1 1 1 1 1 1 1 1 1 1 1 1 1 1 1;],'canBus', '''CAN1''','messageID', [ 402772111;],'idMask', [ 536870911;],'payloadMask', [],'payloadValue', [],'period', [ 0;],'mailbox', '''''','queueSize', [ 1;],'label', [ 0;],'ver', [ 2;],'showID', [ 0;],'showRaw', [ 0;],'showRawMsg', [ 0;],'useStartVals', [ 0;],'extendedId', [ 0;],'showAge', [ 1;],'useSimFunc', [ 0;],'sim_func_name', '''''','fill', [ 0;],'editID', [ 0;],'signalOrder', [ 1;],'signalAscDes', [ 1;],'msgLength', [ 8;])  canBus='CAN1'  mailbox=''  payloadMask=[]  payloadValue=[]  idMask=hex2dec('1FFFFFFF')  queueSize=1  showID=0  label=0  fill=0  id=402772111  showRaw=0  showAge=1  signalOrder=1  signalInfo={{struct('Name', 'DCDC_temperature','StartBit', [ 56;],'SignalSize', [ 8;],'ByteOrder', 'LittleEndian','ValueType', 'SIGNED','Class', 'int8','Signed', [ 1;],'Factor', [ 0.1;],'Offset', [ 0;],'Min', [ 0;],'Max', [ 0;],'Units', 'degC','StartVal', [ 0;],'Comment', 'DCDC temperature','Multiplexed', [ 0;],'Multiplexor', [ 0;],'MultiplexMode_Min', [],'MultiplexMode_Max', []),struct('Name', 'DCDC_outputOverCurrent','StartBit', [ 46;],'SignalSize', [ 1;],'ByteOrder', 'LittleEndian','ValueType', 'UNSIGNED','Class', 'uint8','Signed', [ 0;],'Factor', [ 1;],'Offset', [ 0;],'Min', [ 0;],'Max', [ 0;],'Units', '','StartVal', [ 0;],'Comment', 'DCDC output over current; 0: no error, 1: error','Multiplexed', [ 0;],'Multiplexor', [ 0;],'MultiplexMode_Min', [],'MultiplexMode_Max', []),struct('Name', 'DCDC_outputUnderVoltage','StartBit', [ 45;],'SignalSize', [ 1;],'ByteOrder', 'LittleEndian','ValueType', 'UNSIGNED','Class', 'uint8','Signed', [ 0;],'Factor', [ 1;],'Offset', [ 0;],'Min', [ 0;],'Max', [ 0;],'Units', '','StartVal', [ 0;],'Comment', 'DCDC output under voltage; 0: no error, 1: error','Multiplexed', [ 0;],'Multiplexor', [ 0;],'MultiplexMode_Min', [],'MultiplexMode_Max', []),struct('Name', 'DCDC_outputOverVoltage','StartBit', [ 44;],'SignalSize', [ 1;],'ByteOrder', 'LittleEndian','ValueType', 'UNSIGNED','Class', 'uint8','Signed', [ 0;],'Factor', [ 1;],'Offset', [ 0;],'Min', [ 0;],'Max', [ 0;],'Units', '','StartVal', [ 0;],'Comment', 'DCDC output over voltage; 0: no error, 1: error','Multiplexed', [ 0;],'Multiplexor', [ 0;],'MultiplexMode_Min', [],'MultiplexMode_Max', []),struct('Name', 'DCDC_inputUnderVoltage','StartBit', [ 43;],'SignalSize', [ 1;],'ByteOrder', 'LittleEndian','ValueType', 'UNSIGNED','Class', 'uint8','Signed', [ 0;],'Factor', [ 1;],'Offset', [ 0;],'Min', [ 0;],'Max', [ 0;],'Units', '','StartVal', [ 0;],'Comment', 'DCDC input under voltage; 0: no error, 1: error','Multiplexed', [ 0;],'Multiplexor', [ 0;],'MultiplexMode_Min', [],'MultiplexMode_Max', []),struct('Name', 'DCDC_inputOverVoltage','StartBit', [ 42;],'SignalSize', [ 1;],'ByteOrder', 'LittleEndian','ValueType', 'UNSIGNED','Class', 'uint8','Signed', [ 0;],'Factor', [ 1;],'Offset', [ 0;],'Min', [ 0;],'Max', [ 0;],'Units', '','StartVal', [ 0;],'Comment', 'DCDC input over voltage; 0: no error, 1: error','Multiplexed', [ 0;],'Multiplexor', [ 0;],'MultiplexMode_Min', [],'MultiplexMode_Max', []),struct('Name', 'DCDC_overTempError','StartBit', [ 41;],'SignalSize', [ 1;],'ByteOrder', 'LittleEndian','ValueType', 'UNSIGNED','Class', 'uint8','Signed', [ 0;],'Factor', [ 1;],'Offset', [ 0;],'Min', [ 0;],'Max', [ 0;],'Units', '','StartVal', [ 0;],'Comment', 'DCDC over temp error; 0: no error, 1: error','Multiplexed', [ 0;],'Multiplexor', [ 0;],'MultiplexMode_Min', [],'MultiplexMode_Max', []),struct('Name', 'DCDC_tempWarning','StartBit', [ 40;],'SignalSize', [ 1;],'ByteOrder', 'LittleEndian','ValueType', 'UNSIGNED','Class', 'uint8','Signed', [ 0;],'Factor', [ 1;],'Offset', [ 0;],'Min', [ 0;],'Max', [ 0;],'Units', '','StartVal', [ 0;],'Comment', 'DCDC over temp warning; 0: no warning, 1: warning','Multiplexed', [ 0;],'Multiplexor', [ 0;],'MultiplexMode_Min', [],'MultiplexMode_Max', []),struct('Name', 'DCDC_hvilError','StartBit', [ 39;],'SignalSize', [ 1;],'ByteOrder', 'LittleEndian','ValueType', 'UNSIGNED','Class', 'uint8','Signed', [ 0;],'Factor', [ 1;],'Offset', [ 0;],'Min', [ 0;],'Max', [ 0;],'Units', '','StartVal', [ 0;],'Comment', 'High Voltage Interlock error; 0: no error, 1: error','Multiplexed', [ 0;],'Multiplexor', [ 0;],'MultiplexMode_Min', [],'MultiplexMode_Max', []),struct('Name', 'DCDC_fanControl2','StartBit', [ 38;],'SignalSize', [ 1;],'ByteOrder', 'LittleEndian','ValueType', 'UNSIGNED','Class', 'uint8','Signed', [ 0;],'Factor', [ 1;],'Offset', [ 0;],'Min', [ 0;],'Max', [ 0;],'Units', '','StartVal', [ 0;],'Comment', 'DCDC fan control; 0: off, 1: on','Multiplexed', [ 0;],'Multiplexor', [ 0;],'MultiplexMode_Min', [],'MultiplexMode_Max', []),struct('Name', 'DCDC_shutOffError','StartBit', [ 37;],'SignalSize', [ 1;],'ByteOrder', 'LittleEndian','ValueType', 'UNSIGNED','Class', 'uint8','Signed', [ 0;],'Factor', [ 1;],'Offset', [ 0;],'Min', [ 0;],'Max', [ 0;],'Units', '','StartVal', [ 0;],'Comment', 'DCDC shut off error; 0: no error, 1: error','Multiplexed', [ 0;],'Multiplexor', [ 0;],'MultiplexMode_Min', [],'MultiplexMode_Max', []),struct('Name', 'DCDC_fanControl1','StartBit', [ 36;],'SignalSize', [ 1;],'ByteOrder', 'LittleEndian','ValueType', 'UNSIGNED','Class', 'uint8','Signed', [ 0;],'Factor', [ 1;],'Offset', [ 0;],'Min', [ 0;],'Max', [ 0;],'Units', '','StartVal', [ 0;],'Comment', 'DCDC fan control; 0: off, 1: on','Multiplexed', [ 0;],'Multiplexor', [ 0;],'MultiplexMode_Min', [],'MultiplexMode_Max', []),struct('Name', 'DCDC_canError','StartBit', [ 35;],'SignalSize', [ 1;],'ByteOrder', 'LittleEndian','ValueType', 'UNSIGNED','Class', 'uint8','Signed', [ 0;],'Factor', [ 1;],'Offset', [ 0;],'Min', [ 0;],'Max', [ 0;],'Units', '','StartVal', [ 0;],'Comment', 'DCDC CAN error; 0: no error, 1: error','Multiplexed', [ 0;],'Multiplexor', [ 0;],'MultiplexMode_Min', [],'MultiplexMode_Max', []),struct('Name', 'DCDC_hardwareFault','StartBit', [ 34;],'SignalSize', [ 1;],'ByteOrder', 'LittleEndian','ValueType', 'UNSIGNED','Class', 'uint8','Signed', [ 0;],'Factor', [ 1;],'Offset', [ 0;],'Min', [ 0;],'Max', [ 0;],'Units', '','StartVal', [ 0;],'Comment', 'DCDC hardware error; 0: no error, 1: error','Multiplexed', [ 0;],'Multiplexor', [ 0;],'MultiplexMode_Min', [],'MultiplexMode_Max', []),struct('Name', 'DCDC_status','StartBit', [ 33;],'SignalSize', [ 1;],'ByteOrder', 'LittleEndian','ValueType', 'UNSIGNED','Class', 'uint8','Signed', [ 0;],'Factor', [ 1;],'Offset', [ 0;],'Min', [ 0;],'Max', [ 0;],'Units', '','StartVal', [ 0;],'Comment', 'DCDC state; 0: stopped, 1: working','Multiplexed', [ 0;],'Multiplexor', [ 0;],'MultiplexMode_Min', [],'MultiplexMode_Max', []),struct('Name', 'DCDC_ready','StartBit', [ 32;],'SignalSize', [ 1;],'ByteOrder', 'LittleEndian','ValueType', 'UNSIGNED','Class', 'uint8','Signed', [ 0;],'Factor', [ 1;],'Offset', [ 0;],'Min', [ 0;],'Max', [ 0;],'Units', '','StartVal', [ 0;],'Comment', 'DCDC initialization status; 0: incomplete, 1: complete','Multiplexed', [ 0;],'Multiplexor', [ 0;],'MultiplexMode_Min', [],'MultiplexMode_Max', []),struct('Name', 'DCDC_currentOutput','StartBit', [ 16;],'SignalSize', [ 16;],'ByteOrder', 'LittleEndian','ValueType', 'UNSIGNED','Class', 'uint16','Signed', [ 0;],'Factor', [ 0.1;],'Offset', [ 0;],'Min', [ 0;],'Max', [ 0;],'Units', 'A','StartVal', [ 0;],'Comment', 'DCDC output current','Multiplexed', [ 0;],'Multiplexor', [ 0;],'MultiplexMode_Min', [],'MultiplexMode_Max', []),struct('Name', 'DCDC_voltageOutput','StartBit', [ 0;],'SignalSize', [ 16;],'ByteOrder', 'LittleEndian','ValueType', 'UNSIGNED','Class', 'uint16','Signed', [ 0;],'Factor', [ 0.1;],'Offset', [ 0;],'Min', [ 0;],'Max', [ 0;],'Units', 'V','StartVal', [ 0;],'Comment', 'DCDC output voltage','Multiplexed', [ 0;],'Multiplexor', [ 0;],'MultiplexMode_Min', [],'MultiplexMode_Max', [])}}  showRawMsg=0  useSimFunc=0  sim_func_name=''  useStartVals=0  extendedId=1
      settings: SourceProductName=Raptor
  IO_CAN1_DCDC_Bus : Outport
  wires:
  raptor_can_rxmsg3/13 -> Bus Creator1/13  "DCDC_overTempError"
  raptor_can_rxmsg3/1 -> Bus Creator1/1  "Age"
  raptor_can_rxmsg3/7 -> Bus Creator1/7  "DCDC_hvilError"
  raptor_can_rxmsg3/2 -> Bus Creator1/2  "DCDC_canError"
  raptor_can_rxmsg3/5 -> Bus Creator1/5  "DCDC_fanControl2"
  raptor_can_rxmsg3/18 -> Bus Creator1/18  "DCDC_temperature"
  raptor_can_rxmsg3/14 -> Bus Creator1/14  "DCDC_ready"
  raptor_can_rxmsg3/12 -> Bus Creator1/12  "DCDC_outputUnderVoltage"
  raptor_can_rxmsg3/16 -> Bus Creator1/16  "DCDC_status"
  Bus Creator1/1 -> IO_CAN1_DCDC_Bus/1  "IO_CAN1_DCDC_Bus"
  raptor_can_rxmsg3/8 -> Bus Creator1/8  "DCDC_inputOverVoltage"
  raptor_can_rxmsg3/10 -> Bus Creator1/10  "DCDC_outputOverCurrent"
  raptor_can_rxmsg3/9 -> Bus Creator1/9  "DCDC_inputUnderVoltage"
  raptor_can_rxmsg3/15 -> Bus Creator1/15  "DCDC_shutOffError"
  raptor_can_rxmsg3/11 -> Bus Creator1/11  "DCDC_outputOverVoltage"
  raptor_can_rxmsg3/17 -> Bus Creator1/17  "DCDC_tempWarning"
  raptor_can_rxmsg3/6 -> Bus Creator1/6  "DCDC_hardwarefault"
  raptor_can_rxmsg3/19 -> Bus Creator1/19  "DCDC_voltageOutput"
  raptor_can_rxmsg3/4 -> Bus Creator1/4  "DCDC_fanControl1"
  raptor_can_rxmsg3/3 -> Bus Creator1/3  "DCDC_currentOut"
